simulink subsystem "cabin_suspension"  (R2024a)
settings: Solver=VariableStepAuto  StartTime=0.0  StopTime=10.0  RelTol=1e-3
model mask{Cabin=0}
  mask prompts: Cabin "Cabin Structure"
undefined symbols (not defined in the file or in its folder): cabin, X, Y, Z
libraries: sm_lib x58, Linkage_Shock x16, nesl_utility x6
(part 1 of 2)
settings Model: Creator=lnicolet  LastModifiedBy=lnicolet

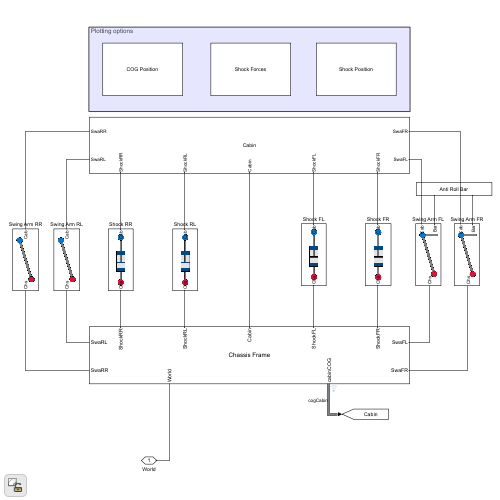
[thumbnail: Simulink's stored preview of the top-level diagram]
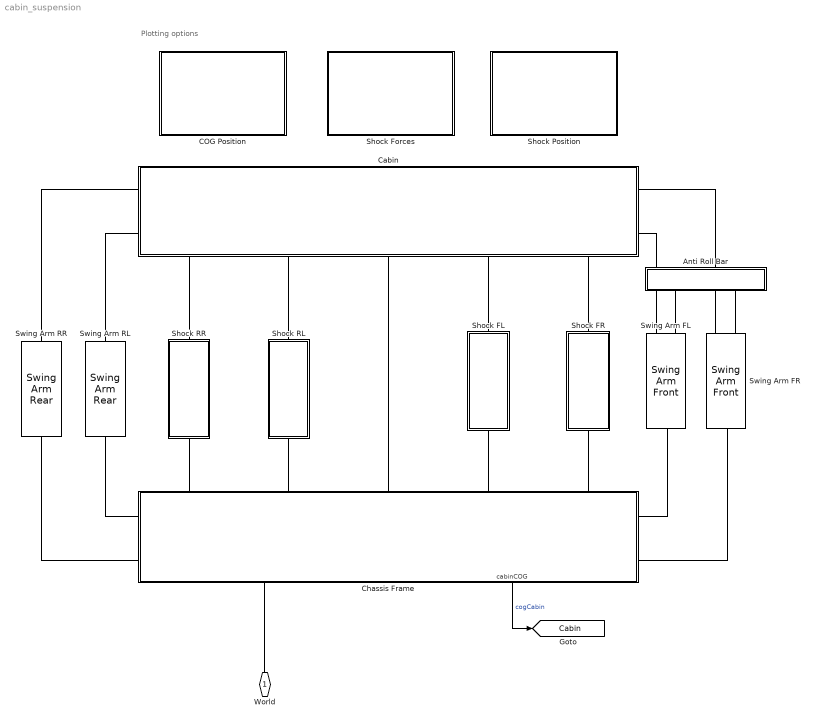
== system cabin_suspension ==
  note: Plotting options
  Anti Roll Bar : Subsystem
      mask Display: disp('Anti Roll Bar')
  COG Position : Subsystem
      settings: OpenFcn=open_system([gcb '/ScopeCabin']);
      mask Display: disp(get_param(gcb,'Name'));
  Cabin : Subsystem
      settings: PortSchema="{\"entries\":[{\"content\":{\"sides\":[{\"content\":{\"connectorIds\":[\"LConn1\",\"LConn2\",\"LConn3\",\"LConn4\",\"LConn5\"]},\"type\":\"ConnectorPlacement.EquallySpacedRectSide\",\"uuid\":\"6c0efb9e-4a15-48d1-a90e-3b8f0520f2fd\"},{\"content\":{\"side\":\"RIGHT\"},\"type\":\"ConnectorPlacement.EquallySpacedRectSide\",\"uuid\":\"c217d90d-c40d-4ab7-8a87-2d7ec4aa75e8\"},{\"content\":{\"connectorIds\":[\"LConn6\",\"LConn7\"],\"side\":\"TOP\"},\"type\":\"ConnectorPlacement.EquallySpacedRectSide\",\"uuid\":\"e70bcc4a-6e95-4530-acee-0e4d1d7170c9\"},{\"content\":{\"connectorIds\":[\"RConn1\",\"RConn2\"],\"side\":\"BOTTOM\"},\"type\":\"ConnectorPlacement.EquallySpacedRectSide\",\"uuid\":\"e953e9a5-e06d-4065-9a29-f0cb41beaf16\"}]},\"type\":\"ConnectorPlacement.EquallySpacedConnector\",\"uuid\":\"c2f1b22e-1df9-453e-a91c-ba57c0256ad1\"}],\"packageUris\":[\"http://schema.mathworks.com/mf0/Connector/R2020b\"],\"version\":\"1.0\"}"
      mask Display: disp('Cabin')
  Chassis Frame : Subsystem
      settings: PortSchema="{\"entries\":[{\"content\":{\"sides\":[{\"content\":{\"connectorIds\":[\"LConn1\",\"Out1\"]},\"type\":\"ConnectorPlacement.EquallySpacedRectSide\",\"uuid\":\"610582a1-14fe-470e-94e3-1e2f1f95b51e\"},{\"content\":{\"connectorIds\":[\"RConn1\",\"RConn2\",\"RConn3\",\"RConn4\",\"RConn5\"],\"side\":\"RIGHT\"},\"type\":\"ConnectorPlacement.EquallySpacedRectSide\",\"uuid\":\"a77f2f37-ea81-4a54-9e68-b60d989bebab\"},{\"content\":{\"connectorIds\":[\"LConn2\",\"LConn3\"],\"side\":\"TOP\"},\"type\":\"ConnectorPlacement.EquallySpacedRectSide\",\"uuid\":\"50ec98b4-a561-4ba0-8e8b-a43aa9d2b054\"},{\"content\":{\"connectorIds\":[\"RConn6\",\"RConn7\"],\"side\":\"BOTTOM\"},\"type\":\"ConnectorPlacement.EquallySpacedRectSide\",\"uuid\":\"9dd61552-a50f-4419-91a1-3a5b07471613\"}]},\"type\":\"ConnectorPlacement.EquallySpacedConnector\",\"uuid\":\"113db540-2e6d-4d54-be76-d99676ae8778\"}],\"packageUris\":[\"http://schema.mathworks.com/mf0/Connector/R2020b\"],\"version\":\"1.0\"}"
      mask Display: disp('Chassis Frame')
  Shock FL : Subsystem
      mask Display: image('Shock_Assembly_IMAGE.png');
  Shock FR : Subsystem
      mask Display: image('Shock_Assembly_IMAGE.png');
  Shock Forces : Subsystem
      settings: OpenFcn=open_system([gcb '/ScopeForces']);
      mask Display: disp(get_param(gcb,'Name'));
  Shock Position : Subsystem
      settings: OpenFcn=open_system([gcb '/ScopeDef']);
      mask Display: disp(get_param(gcb,'Name'));
  Shock RL : Subsystem
      mask Display: image('Shock_Assembly_IMAGE.png');
  Shock RR : Subsystem
      mask Display: image('Shock_Assembly_IMAGE.png');
  Swing Arm FL : Linkage_Shock/Swing Arm Front  posCab=cabin.swingArmCabFL  posCha=cabin.swingArmChasFL  azimuth=cabin.azimuthFL  elevation=cabin.elevationFL
  Swing Arm FR : Linkage_Shock/Swing Arm Front  posCab=cabin.swingArmCabFR  posCha=cabin.swingArmChasFR  azimuth=cabin.azimuthFR  elevation=cabin.elevationFR
  Swing Arm RL : Linkage_Shock/Swing Arm Rear  posCab=cabin.swingArmCabRL  posCha=cabin.swingArmChasRL
  Swing Arm RR : Linkage_Shock/Swing Arm Rear  posCab=cabin.swingArmCabRR  posCha=cabin.swingArmChasRR
  World : PMIOPort  Side=Left
  tag scope: Cabin=global
  wires:
  Chassis Frame/1(cabinCOG) -> [Cabin]  "cogCabin"
  connections:
  Cabin/LConn2 -- Shock RL/RConn1
  Swing Arm RL/LConn1 -- Chassis Frame/LConn3
  World/RConn1 -- Chassis Frame/LConn1
  Swing Arm FR/LConn1 -- Chassis Frame/RConn6
  Chassis Frame/RConn3 -- Cabin/LConn3
  Cabin/LConn1 -- Shock RR/RConn1
  Swing Arm FL/LConn1 -- Chassis Frame/RConn7
  Swing Arm FL/RConn1 -- Cabin/RConn1
  Cabin/LConn4 -- Shock FL/RConn1
  Swing Arm FR/RConn1 -- Cabin/RConn2
  Chassis Frame/LConn2 -- Swing Arm RR/LConn1
  Chassis Frame/RConn4 -- Shock FL/LConn1
  Swing Arm RR/RConn1 -- Cabin/LConn7
  Chassis Frame/RConn5 -- Shock FR/LConn1
  Swing Arm RL/RConn1 -- Cabin/LConn6
  Cabin/LConn5 -- Shock FR/RConn1
  Swing Arm FL/RConn2 -- Anti Roll Bar/LConn1
  Chassis Frame/RConn2 -- Shock RL/LConn1
  Chassis Frame/RConn1 -- Shock RR/LConn1
  Swing Arm FR/RConn2 -- Anti Roll Bar/LConn2

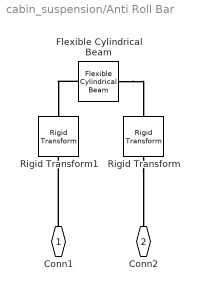
== system cabin_suspension/Anti Roll Bar ==
  Flexible Cylindrical Beam : sm_lib/Body Elements/Flexible Bodies/Beams/Flexible Cylindrical Beam  SectionType=Hollow  Radius=cabin.antiRollBarRadiusOut  RadiusUnits=m  Thickness=cabin.antiRollBarRadiusOut-cabin.antiRollBarRadiusInn  ThicknessUnits=m  Length=norm(cabin.swingArmCabFR-cabin.swingArmCabFL);  LengthUnits=m  StiffnessAndInertiaType=CalculateFromGeometry  Density=cabin.antiRollBarDensity  DensityUnits=kg/m^3  ModuliType=YoungsPoissons  YoungsModulus=cabin.antiRollBarEModulus  YoungsModulusUnits=GPa  PoissonsRatio=cabin.antiRollBarPoisson  ShearModulus=26  ShearModulusUnits=GPa  GeometricCentroid=[0 0]  GeometricCentroidUnits=m  BendingCentroid=[0 0]  BendingCentroidUnits=m  ShearCenter=[0 0]  ShearCenterUnits=m  AxialRigidity=1  AxialRigidityUnits=Pa*m^2  FlexuralRigidity=[1 1]  FlexuralRigidityUnits=Pa*m^4  CrossFlexuralRigidity=0  CrossFlexuralRigidityUnits=Pa*m^4  TorsionalRigidity=1  TorsionalRigidityUnits=Pa*m^4  CenterOfMass=[0 0]  CenterOfMassUnits=m  MassPerUnitLength=1  MassPerUnitLengthUnits=kg/m  MassMomentOfInertiaDensity=[1 1]  MassMomentOfInertiaDensityUnits=kg*m  MassProductOfInertiaDensity=0  MassProductOfInertiaDensityUnits=kg*m  DampingType=Proportional  ProportionalDampingAlpha=0  ProportionalDampingAlphaUnits=1/s  ProportionalDampingBeta=0.001  ProportionalDampingBetaUnits=s  UniformModalDampingRatio=0.01  NumElements=1  ReductionType=None  NumRetainedModes=1  GraphicType=FromGeometry  GraphicVisPropType=SimpleVisualProperties  GraphicDiffuseColor=[0.5 0.5 0.5]  GraphicOpacity=1  GraphicSpecularColor=[0.5 0.5 0.5 1.0]  GraphicAmbientColor=[0.15 0.15 0.15 1.0]  GraphicEmissiveColor=[0.0 0.0 0.0 1.0]  GraphicShininess=75  DoExposeZminFrame=on  DoExposeZmaxFrame=on  SerializedFrames=<Frames/>
  Rigid Transform : sm_lib/Frames and Transforms/Rigid Transform  RotationMethod=StandardAxis  FollAlignAxisA=+X  BaseAlignAxisA=+Y  FollAlignAxisB=+Y  BaseAlignAxisB=+Z  RotationStandardAxis=+X  RotationAngle=90  RotationAngleUnits=deg  RotationArbitraryAxis=[0 0 1]  RotationSequenceAxes=FollowerAxes  RotationSequence=XYX  RotationSequenceAngles=[0 0 0]  RotationSequenceAnglesUnits=deg  RotationMatrix=[1 0 0;0 1 0;0 0 1]  Quaternion=[1 0 0 0]  TranslationMethod=None  TranslationCartesianOffset=[0 0 0]  TranslationCartesianOffsetUnits=m  TranslationStandardAxis=+Z  TranslationStandardOffset=0  TranslationStandardOffsetUnits=m  TranslationROffset=0  TranslationROffsetUnits=m  TranslationThetaOffset=0  TranslationThetaOffsetUnits=deg  TranslationZOffset=0  TranslationZOffsetUnits=m
  Rigid Transform1 : sm_lib/Frames and Transforms/Rigid Transform  RotationMethod=StandardAxis  FollAlignAxisA=+X  BaseAlignAxisA=+Y  FollAlignAxisB=+Y  BaseAlignAxisB=+Z  RotationStandardAxis=+X  RotationAngle=90  RotationAngleUnits=deg  RotationArbitraryAxis=[0 0 1]  RotationSequenceAxes=FollowerAxes  RotationSequence=XYX  RotationSequenceAngles=[0 0 0]  RotationSequenceAnglesUnits=deg  RotationMatrix=[1 0 0;0 1 0;0 0 1]  Quaternion=[1 0 0 0]  TranslationMethod=None  TranslationCartesianOffset=[0 0 0]  TranslationCartesianOffsetUnits=m  TranslationStandardAxis=+Z  TranslationStandardOffset=0  TranslationStandardOffsetUnits=m  TranslationROffset=0  TranslationROffsetUnits=m  TranslationThetaOffset=0  TranslationThetaOffsetUnits=deg  TranslationZOffset=0  TranslationZOffsetUnits=m
  Conn1 : PMIOPort  Side=Left
  Conn2 : PMIOPort  Port=2  Side=Left
  connections:
  Conn1/RConn1 -- Rigid Transform1/LConn1
  Flexible Cylindrical Beam/RConn1 -- Rigid Transform/RConn1
  Rigid Transform/LConn1 -- Conn2/RConn1
  Flexible Cylindrical Beam/LConn1 -- Rigid Transform1/RConn1

== system cabin_suspension/COG Position ==
  Bus Selector : BusSelector  OutputSignals=px,py,pz,angx,angy,angz
  ScopeCabin : Scope  NumInputPorts=6
  wires:
  Bus Selector/6 -> ScopeCabin/6  "<angz>"
  Bus Selector/5 -> ScopeCabin/5  "<angy>"
  Bus Selector/4 -> ScopeCabin/4  "<angx>"
  Bus Selector/3 -> ScopeCabin/3  "<pz>"
  Bus Selector/2 -> ScopeCabin/2  "<py>"
  Bus Selector/1 -> ScopeCabin/1  "<px>"
  [Cabin] -> Bus Selector/1

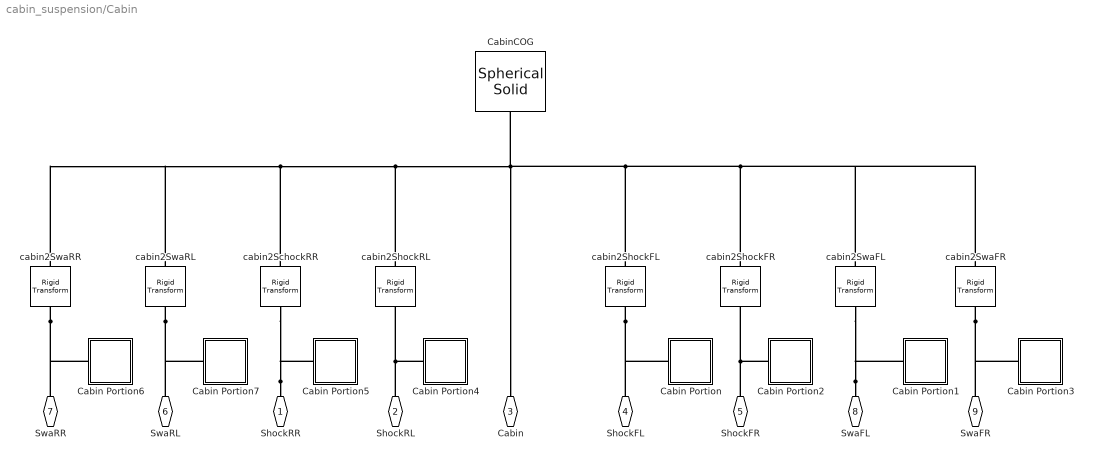
== system cabin_suspension/Cabin ==
  Cabin Portion : Subsystem
  Cabin Portion1 : Subsystem
  Cabin Portion2 : Subsystem
  Cabin Portion3 : Subsystem
  Cabin Portion4 : Subsystem
  Cabin Portion5 : Subsystem
  Cabin Portion6 : Subsystem
  Cabin Portion7 : Subsystem
  CabinCOG : sm_lib/Body Elements/Spherical Solid  SphereRadius=0.03  SphereRadiusUnits=m  ExportEntireGeometry=off  InertiaType=Custom  BasedOnType=Mass  Density=1000  DensityUnits=kg/m^3  Mass=cabin.cabinMass  MassUnits=kg  CenterOfMass=[0 0 0]  CenterOfMassUnits=m  MomentsOfInertia=[cabin.cabinJxx,cabin.cabinJyy,cabin.cabinJzz]  MomentsOfInertiaUnits=kg*m^2  ProductsOfInertia=[0 0 0]  ProductsOfInertiaUnits=kg*m^2  GraphicType=FromGeometry  MarkerShape=Sphere  MarkerSize=10  GraphicVisPropType=SimpleVisualProperties  GraphicDiffuseColor=[0,0,1]  GraphicOpacity=1  GraphicSpecularColor=[0.5 0.5 0.5 1.0]  GraphicAmbientColor=[0.15 0.15 0.15 1.0]  GraphicEmissiveColor=[0.0 0.0 0.0 1.0]  GraphicShininess=75  DoExposeReferenceFrame=on  SerializedFrames=<Frames/>
  cabin2SchockRR : sm_lib/Frames and Transforms/Rigid Transform  RotationMethod=None  FollAlignAxisA=+X  BaseAlignAxisA=+Y  FollAlignAxisB=+Y  BaseAlignAxisB=+Z  RotationStandardAxis=+Z  RotationAngle=0  RotationAngleUnits=deg  RotationArbitraryAxis=[0 0 1]  RotationSequenceAxes=FollowerAxes  RotationSequence=XYX  RotationSequenceAngles=[0 0 0]  RotationSequenceAnglesUnits=deg  RotationMatrix=[1 0 0;0 1 0;0 0 1]  Quaternion=[1 0 0 0]  TranslationMethod=Cartesian  TranslationCartesianOffset=cabin.schockTopPosRR-cabin.cabinOriginStart  TranslationCartesianOffsetUnits=m  TranslationStandardAxis=+Z  TranslationStandardOffset=0  TranslationStandardOffsetUnits=m  TranslationROffset=0  TranslationROffsetUnits=m  TranslationThetaOffset=0  TranslationThetaOffsetUnits=deg  TranslationZOffset=0  TranslationZOffsetUnits=m
  cabin2ShockFL : sm_lib/Frames and Transforms/Rigid Transform  RotationMethod=None  FollAlignAxisA=+X  BaseAlignAxisA=+Y  FollAlignAxisB=+Y  BaseAlignAxisB=+Z  RotationStandardAxis=+Z  RotationAngle=0  RotationAngleUnits=deg  RotationArbitraryAxis=[0 0 1]  RotationSequenceAxes=FollowerAxes  RotationSequence=XYX  RotationSequenceAngles=[0 0 0]  RotationSequenceAnglesUnits=deg  RotationMatrix=[1 0 0;0 1 0;0 0 1]  Quaternion=[1 0 0 0]  TranslationMethod=Cartesian  TranslationCartesianOffset=cabin.schockTopPosFL-cabin.cabinOriginStart  TranslationCartesianOffsetUnits=m  TranslationStandardAxis=+Z  TranslationStandardOffset=0  TranslationStandardOffsetUnits=m  TranslationROffset=0  TranslationROffsetUnits=m  TranslationThetaOffset=0  TranslationThetaOffsetUnits=deg  TranslationZOffset=0  TranslationZOffsetUnits=m
  cabin2ShockFR : sm_lib/Frames and Transforms/Rigid Transform  RotationMethod=None  FollAlignAxisA=+X  BaseAlignAxisA=+Y  FollAlignAxisB=+Y  BaseAlignAxisB=+Z  RotationStandardAxis=+Z  RotationAngle=0  RotationAngleUnits=deg  RotationArbitraryAxis=[0 0 1]  RotationSequenceAxes=FollowerAxes  RotationSequence=XYX  RotationSequenceAngles=[0 0 0]  RotationSequenceAnglesUnits=deg  RotationMatrix=[1 0 0;0 1 0;0 0 1]  Quaternion=[1 0 0 0]  TranslationMethod=Cartesian  TranslationCartesianOffset=cabin.schockTopPosFR-cabin.cabinOriginStart  TranslationCartesianOffsetUnits=m  TranslationStandardAxis=+Z  TranslationStandardOffset=0  TranslationStandardOffsetUnits=m  TranslationROffset=0  TranslationROffsetUnits=m  TranslationThetaOffset=0  TranslationThetaOffsetUnits=deg  TranslationZOffset=0  TranslationZOffsetUnits=m
  cabin2ShockRL : sm_lib/Frames and Transforms/Rigid Transform  RotationMethod=None  FollAlignAxisA=+X  BaseAlignAxisA=+Y  FollAlignAxisB=+Y  BaseAlignAxisB=+Z  RotationStandardAxis=+Z  RotationAngle=0  RotationAngleUnits=deg  RotationArbitraryAxis=[0 0 1]  RotationSequenceAxes=FollowerAxes  RotationSequence=XYX  RotationSequenceAngles=[0 0 0]  RotationSequenceAnglesUnits=deg  RotationMatrix=[1 0 0;0 1 0;0 0 1]  Quaternion=[1 0 0 0]  TranslationMethod=Cartesian  TranslationCartesianOffset=cabin.schockTopPosRL-cabin.cabinOriginStart  TranslationCartesianOffsetUnits=m  TranslationStandardAxis=+Z  TranslationStandardOffset=0  TranslationStandardOffsetUnits=m  TranslationROffset=0  TranslationROffsetUnits=m  TranslationThetaOffset=0  TranslationThetaOffsetUnits=deg  TranslationZOffset=0  TranslationZOffsetUnits=m
  cabin2SwaFL : sm_lib/Frames and Transforms/Rigid Transform  RotationMethod=None  FollAlignAxisA=+X  BaseAlignAxisA=+Y  FollAlignAxisB=+Y  BaseAlignAxisB=+Z  RotationStandardAxis=+X  RotationAngle=-90  RotationAngleUnits=deg  RotationArbitraryAxis=[0 0 1]  RotationSequenceAxes=FollowerAxes  RotationSequence=XYX  RotationSequenceAngles=[0 0 0]  RotationSequenceAnglesUnits=deg  RotationMatrix=[1 0 0;0 1 0;0 0 1]  Quaternion=[1 0 0 0]  TranslationMethod=Cartesian  TranslationCartesianOffset=cabin.swingArmCabFL-cabin.cabinOriginStart  TranslationCartesianOffsetUnits=m  TranslationStandardAxis=+Z  TranslationStandardOffset=0  TranslationStandardOffsetUnits=m  TranslationROffset=0  TranslationROffsetUnits=m  TranslationThetaOffset=0  TranslationThetaOffsetUnits=deg  TranslationZOffset=0  TranslationZOffsetUnits=m
  cabin2SwaFR : sm_lib/Frames and Transforms/Rigid Transform  RotationMethod=None  FollAlignAxisA=+X  BaseAlignAxisA=+Y  FollAlignAxisB=+Y  BaseAlignAxisB=+Z  RotationStandardAxis=+X  RotationAngle=-90  RotationAngleUnits=deg  RotationArbitraryAxis=[0 0 1]  RotationSequenceAxes=FollowerAxes  RotationSequence=XYX  RotationSequenceAngles=[0 0 0]  RotationSequenceAnglesUnits=deg  RotationMatrix=[1 0 0;0 1 0;0 0 1]  Quaternion=[1 0 0 0]  TranslationMethod=Cartesian  TranslationCartesianOffset=cabin.swingArmCabFR-cabin.cabinOriginStart  TranslationCartesianOffsetUnits=m  TranslationStandardAxis=+Z  TranslationStandardOffset=0  TranslationStandardOffsetUnits=m  TranslationROffset=0  TranslationROffsetUnits=m  TranslationThetaOffset=0  TranslationThetaOffsetUnits=deg  TranslationZOffset=0  TranslationZOffsetUnits=m
  cabin2SwaRL : sm_lib/Frames and Transforms/Rigid Transform  RotationMethod=None  FollAlignAxisA=+X  BaseAlignAxisA=+Y  FollAlignAxisB=+Y  BaseAlignAxisB=+Z  RotationStandardAxis=+X  RotationAngle=-90  RotationAngleUnits=deg  RotationArbitraryAxis=[0 0 1]  RotationSequenceAxes=FollowerAxes  RotationSequence=XYX  RotationSequenceAngles=[0 0 0]  RotationSequenceAnglesUnits=deg  RotationMatrix=[1 0 0;0 1 0;0 0 1]  Quaternion=[1 0 0 0]  TranslationMethod=Cartesian  TranslationCartesianOffset=cabin.swingArmCabRL-cabin.cabinOriginStart  TranslationCartesianOffsetUnits=m  TranslationStandardAxis=+Z  TranslationStandardOffset=0  TranslationStandardOffsetUnits=m  TranslationROffset=0  TranslationROffsetUnits=m  TranslationThetaOffset=0  TranslationThetaOffsetUnits=deg  TranslationZOffset=0  TranslationZOffsetUnits=m
  cabin2SwaRR : sm_lib/Frames and Transforms/Rigid Transform  RotationMethod=None  FollAlignAxisA=+X  BaseAlignAxisA=+Y  FollAlignAxisB=+Y  BaseAlignAxisB=+Z  RotationStandardAxis=+X  RotationAngle=-90  RotationAngleUnits=deg  RotationArbitraryAxis=[0 0 1]  RotationSequenceAxes=FollowerAxes  RotationSequence=XYX  RotationSequenceAngles=[0 0 0]  RotationSequenceAnglesUnits=deg  RotationMatrix=[1 0 0;0 1 0;0 0 1]  Quaternion=[1 0 0 0]  TranslationMethod=Cartesian  TranslationCartesianOffset=cabin.swingArmCabRR-cabin.cabinOriginStart  TranslationCartesianOffsetUnits=m  TranslationStandardAxis=+Z  TranslationStandardOffset=0  TranslationStandardOffsetUnits=m  TranslationROffset=0  TranslationROffsetUnits=m  TranslationThetaOffset=0  TranslationThetaOffsetUnits=deg  TranslationZOffset=0  TranslationZOffsetUnits=m
  ShockRR : PMIOPort  Side=Left
  ShockRL : PMIOPort  Port=2  Side=Left
  Cabin : PMIOPort  Port=3  Side=Left
  ShockFL : PMIOPort  Port=4  Side=Left
  ShockFR : PMIOPort  Port=5  Side=Left
  SwaRL : PMIOPort  Port=6  Side=Left
  SwaRR : PMIOPort  Port=7  Side=Left
  SwaFL : PMIOPort  Port=8  Side=Right
  SwaFR : PMIOPort  Port=9  Side=Right
  connections:
  SwaFL/RConn1 -- Cabin Portion1/LConn1 -- cabin2SwaFL/RConn1
  cabin2SwaFR/RConn1 -- Cabin Portion3/LConn1 -- SwaFR/RConn1
  cabin2ShockFL/RConn1 -- Cabin Portion/LConn1 -- ShockFL/RConn1
  cabin2SwaRR/RConn1 -- Cabin Portion6/LConn1 -- SwaRR/RConn1
  ShockRR/RConn1 -- Cabin Portion5/LConn1 -- cabin2SchockRR/RConn1
  cabin2SwaRL/RConn1 -- Cabin Portion7/LConn1 -- SwaRL/RConn1
  Cabin Portion2/LConn1 -- cabin2ShockFR/RConn1 -- ShockFR/RConn1
  Cabin Portion4/LConn1 -- cabin2ShockRL/RConn1 -- ShockRL/RConn1
  cabin2ShockFL/LConn1 -- cabin2SchockRR/LConn1 -- cabin2SwaRR/LConn1 -- cabin2SwaRL/LConn1 -- cabin2ShockRL/LConn1 -- Cabin/RConn1 -- CabinCOG/RConn1 -- cabin2ShockFR/LConn1 -- cabin2SwaFR/LConn1 -- cabin2SwaFL/LConn1

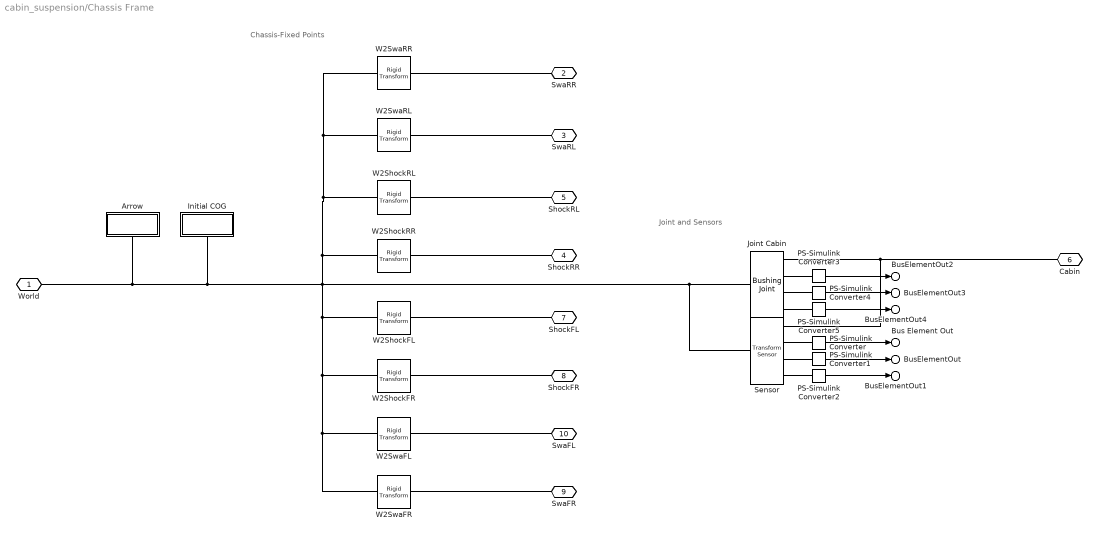
== system cabin_suspension/Chassis Frame ==
  note: Joint and Sensors
  note: Chassis-Fixed Points
  Arrow : Subsystem
      mask Display: disp(get_param(gcb,'Name'));
  Initial COG : Subsystem
      mask Display: disp(get_param(gcb,'Name'));
  Joint Cabin : sm_lib/Joints/Bushing Joint  JointMode=Normal  CompositeWrenchDir=FollowerOnBase  CompositeWrenchFrame=BaseFrame  SenseConstraintForce=off  SenseConstraintTorque=off  SenseTotalForce=off  SenseTotalTorque=off  PxPositionTargetSpecify=on  PxPositionTargetPriority=High  PxPositionTargetValue=cabin.cabinOriginStart(1)  PxPositionTargetValueUnits=m  PxVelocityTargetSpecify=off  PxVelocityTargetPriority=High  PxVelocityTargetValue=0  PxVelocityTargetValueUnits=m/s  PxEquilibriumPosition=0  PxEquilibriumPositionUnits=m  PxSpringStiffness=0  PxSpringStiffnessUnits=N/m  PxDampingCoefficient=0  PxDampingCoefficientUnits=N/(m/s)  PxLowerLimitSpecify=off  PxLowerLimitBound=-1  PxLowerLimitBoundUnits=m  PxLowerLimitStiffness=1e6  PxLowerLimitStiffnessUnits=N/m  PxLowerLimitDamping=1e3  PxLowerLimitDampingUnits=N/(m/s)  PxLowerLimitTransitionRegionWidth=1e-4  PxLowerLimitTransitionRegionWidthUnits=m  PxUpperLimitSpecify=off  PxUpperLimitBound=1  PxUpperLimitBoundUnits=m  PxUpperLimitStiffness=1e6  PxUpperLimitStiffnessUnits=N/m  PxUpperLimitDamping=1e3  PxUpperLimitDampingUnits=N/(m/s)  PxUpperLimitTransitionRegionWidth=1e-4  PxUpperLimitTransitionRegionWidthUnits=m  PxTorqueActuationMode=NoTorque  PxMotionActuationMode=ComputedMotion  PxSensePosition=off  PxSenseVelocity=off  PxSenseAcceleration=off  PxSenseTorqueForce=off  PxSenseLowerLimitTorqueForce=off  PxSenseUpperLimitTorqueForce=off  PyPositionTargetSpecify=on  PyPositionTargetPriority=High  PyPositionTargetValue=cabin.cabinOriginStart(2)  PyPositionTargetValueUnits=m  PyVelocityTargetSpecify=off  PyVelocityTargetPriority=High  PyVelocityTargetValue=0  PyVelocityTargetValueUnits=m/s  PyEquilibriumPosition=0  PyEquilibriumPositionUnits=m  PySpringStiffness=0  PySpringStiffnessUnits=N/m  PyDampingCoefficient=0  PyDampingCoefficientUnits=N/(m/s)  PyLowerLimitSpecify=off  PyLowerLimitBound=-1  PyLowerLimitBoundUnits=m  PyLowerLimitStiffness=1e6  PyLowerLimitStiffnessUnits=N/m  PyLowerLimitDamping=1e3  PyLowerLimitDampingUnits=N/(m/s)  PyLowerLimitTransitionRegionWidth=1e-4  PyLowerLimitTransitionRegionWidthUnits=m  PyUpperLimitSpecify=off  PyUpperLimitBound=1  PyUpperLimitBoundUnits=m  PyUpperLimitStiffness=1e6  PyUpperLimitStiffnessUnits=N/m  PyUpperLimitDamping=1e3  PyUpperLimitDampingUnits=N/(m/s)  PyUpperLimitTransitionRegionWidth=1e-4  PyUpperLimitTransitionRegionWidthUnits=m  PyTorqueActuationMode=NoTorque  PyMotionActuationMode=ComputedMotion  PySensePosition=off  PySenseVelocity=off  PySenseAcceleration=off  PySenseTorqueForce=off  PySenseLowerLimitTorqueForce=off  PySenseUpperLimitTorqueForce=off  PzPositionTargetSpecify=on  PzPositionTargetPriority=High  PzPositionTargetValue=cabin.cabinOriginStart(3)  PzPositionTargetValueUnits=m  PzVelocityTargetSpecify=off  PzVelocityTargetPriority=High  PzVelocityTargetValue=0  PzVelocityTargetValueUnits=m/s  PzEquilibriumPosition=0  PzEquilibriumPositionUnits=m  PzSpringStiffness=0  PzSpringStiffnessUnits=N/m  PzDampingCoefficient=0  PzDampingCoefficientUnits=N/(m/s)  PzLowerLimitSpecify=off  PzLowerLimitBound=-1  PzLowerLimitBoundUnits=m  PzLowerLimitStiffness=1e6  PzLowerLimitStiffnessUnits=N/m  PzLowerLimitDamping=1e3  PzLowerLimitDampingUnits=N/(m/s)  PzLowerLimitTransitionRegionWidth=1e-4  PzLowerLimitTransitionRegionWidthUnits=m  PzUpperLimitSpecify=off  PzUpperLimitBound=1  PzUpperLimitBoundUnits=m  PzUpperLimitStiffness=1e6  PzUpperLimitStiffnessUnits=N/m  PzUpperLimitDamping=1e3  PzUpperLimitDampingUnits=N/(m/s)  PzUpperLimitTransitionRegionWidth=1e-4  PzUpperLimitTransitionRegionWidthUnits=m  PzTorqueActuationMode=NoTorque  PzMotionActuationMode=ComputedMotion  PzSensePosition=off  PzSenseVelocity=off  PzSenseAcceleration=off  PzSenseTorqueForce=off  PzSenseLowerLimitTorqueForce=off  PzSenseUpperLimitTorqueForce=off  RxPositionTargetSpecify=on  RxPositionTargetPriority=High  RxPositionTargetValue=0  RxPositionTargetValueUnits=deg  RxVelocityTargetSpecify=off  RxVelocityTargetPriority=High  RxVelocityTargetValue=0  RxVelocityTargetValueUnits=deg/s  RxEquilibriumPosition=0  RxEquilibriumPositionUnits=deg  RxSpringStiffness=0  RxSpringStiffnessUnits=N*m/deg  RxDampingCoefficient=0  RxDampingCoefficientUnits=N*m/(deg/s)  RxLowerLimitSpecify=off  RxLowerLimitBound=-90  RxLowerLimitBoundUnits=deg  RxLowerLimitStiffness=1e4  RxLowerLimitStiffnessUnits=N*m/deg  RxLowerLimitDamping=10  RxLowerLimitDampingUnits=N*m/(deg/s)  RxLowerLimitTransitionRegionWidth=0.1  RxLowerLimitTransitionRegionWidthUnits=deg  RxUpperLimitSpecify=off  RxUpperLimitBound=90  RxUpperLimitBoundUnits=deg  RxUpperLimitStiffness=1e4  RxUpperLimitStiffnessUnits=N*m/deg  RxUpperLimitDamping=10  RxUpperLimitDampingUnits=N*m/(deg/s)  RxUpperLimitTransitionRegionWidth=0.1  RxUpperLimitTransitionRegionWidthUnits=deg  RxTorqueActuationMode=NoTorque  RxMotionActuationMode=ComputedMotion  RxSensePosition=on  RxSenseVelocity=off  RxSenseAcceleration=off  RxSenseTorqueForce=off  RxSenseLowerLimitTorqueForce=off  RxSenseUpperLimitTorqueForce=off  RyPositionTargetSpecify=on  RyPositionTargetPriority=High  RyPositionTargetValue=0  RyPositionTargetValueUnits=deg  RyVelocityTargetSpecify=off  RyVelocityTargetPriority=High  RyVelocityTargetValue=0  RyVelocityTargetValueUnits=deg/s  RyEquilibriumPosition=0  RyEquilibriumPositionUnits=deg  RySpringStiffness=0  RySpringStiffnessUnits=N*m/deg  RyDampingCoefficient=0  RyDampingCoefficientUnits=N*m/(deg/s)  RyLowerLimitSpecify=off  RyLowerLimitBound=-90  RyLowerLimitBoundUnits=deg  RyLowerLimitStiffness=1e4  RyLowerLimitStiffnessUnits=N*m/deg  RyLowerLimitDamping=10  RyLowerLimitDampingUnits=N*m/(deg/s)  RyLowerLimitTransitionRegionWidth=0.1  RyLowerLimitTransitionRegionWidthUnits=deg  RyUpperLimitSpecify=off  RyUpperLimitBound=90  RyUpperLimitBoundUnits=deg  RyUpperLimitStiffness=1e4  RyUpperLimitStiffnessUnits=N*m/deg  RyUpperLimitDamping=10  RyUpperLimitDampingUnits=N*m/(deg/s)  RyUpperLimitTransitionRegionWidth=0.1  RyUpperLimitTransitionRegionWidthUnits=deg  RyTorqueActuationMode=NoTorque  RyMotionActuationMode=ComputedMotion  RySensePosition=on  RySenseVelocity=off  RySenseAcceleration=off  RySenseTorqueForce=off  RySenseLowerLimitTorqueForce=off  RySenseUpperLimitTorqueForce=off  RzPositionTargetSpecify=on  RzPositionTargetPriority=High  RzPositionTargetValue=0  RzPositionTargetValueUnits=deg  RzVelocityTargetSpecify=off  RzVelocityTargetPriority=High  RzVelocityTargetValue=0  RzVelocityTargetValueUnits=deg/s  RzEquilibriumPosition=0  RzEquilibriumPositionUnits=deg  RzSpringStiffness=0  RzSpringStiffnessUnits=N*m/deg  RzDampingCoefficient=0  RzDampingCoefficientUnits=N*m/(deg/s)  RzLowerLimitSpecify=off  RzLowerLimitBound=-90  RzLowerLimitBoundUnits=deg  RzLowerLimitStiffness=1e4  RzLowerLimitStiffnessUnits=N*m/deg  RzLowerLimitDamping=10  RzLowerLimitDampingUnits=N*m/(deg/s)  RzLowerLimitTransitionRegionWidth=0.1  RzLowerLimitTransitionRegionWidthUnits=deg  RzUpperLimitSpecify=off  RzUpperLimitBound=90  RzUpperLimitBoundUnits=deg  RzUpperLimitStiffness=1e4  RzUpperLimitStiffnessUnits=N*m/deg  RzUpperLimitDamping=10  RzUpperLimitDampingUnits=N*m/(deg/s)  RzUpperLimitTransitionRegionWidth=0.1  RzUpperLimitTransitionRegionWidthUnits=deg  RzTorqueActuationMode=NoTorque  RzMotionActuationMode=ComputedMotion  RzSensePosition=on  RzSenseVelocity=off  RzSenseAcceleration=off  RzSenseTorqueForce=off  RzSenseLowerLimitTorqueForce=off  RzSenseUpperLimitTorqueForce=off
  PS-Simulink Converter : nesl_utility/PS-Simulink Converter  PhysicalDomain=network_engine_domain  SubClassName=ps_output  LeftPortType=input  RightPortType=output  PseudoPeriodic=off  Frequencies=[]  VectorFormat=inherit  Unit=m  AffineConversion=off
  PS-Simulink Converter1 : nesl_utility/PS-Simulink Converter  PhysicalDomain=network_engine_domain  SubClassName=ps_output  LeftPortType=input  RightPortType=output  PseudoPeriodic=off  Frequencies=[]  VectorFormat=inherit  Unit=m  AffineConversion=off
  PS-Simulink Converter2 : nesl_utility/PS-Simulink Converter  PhysicalDomain=network_engine_domain  SubClassName=ps_output  LeftPortType=input  RightPortType=output  PseudoPeriodic=off  Frequencies=[]  VectorFormat=inherit  Unit=m  AffineConversion=off
  PS-Simulink Converter3 : nesl_utility/PS-Simulink Converter  PhysicalDomain=network_engine_domain  SubClassName=ps_output  LeftPortType=input  RightPortType=output  PseudoPeriodic=off  Frequencies=[]  VectorFormat=inherit  Unit=deg  AffineConversion=off
  PS-Simulink Converter4 : nesl_utility/PS-Simulink Converter  PhysicalDomain=network_engine_domain  SubClassName=ps_output  LeftPortType=input  RightPortType=output  PseudoPeriodic=off  Frequencies=[]  VectorFormat=inherit  Unit=deg  AffineConversion=off
  PS-Simulink Converter5 : nesl_utility/PS-Simulink Converter  PhysicalDomain=network_engine_domain  SubClassName=ps_output  LeftPortType=input  RightPortType=output  PseudoPeriodic=off  Frequencies=[]  VectorFormat=inherit  Unit=deg  AffineConversion=off
  "Sensor " : sm_lib/Frames and Transforms/Transform Sensor  MeasurementFrame=World  RotationSequence=XYX  SenseAngle=off  SenseAxis=off  SenseQ=off  SenseR=off  SenseRotationSequence=off  SenseOmegaX=off  SenseOmegaY=off  SenseOmegaZ=off  SenseOmega=off  SenseQDot=off  SenseRDot=off  SenseRotationSequenceDot=off  SenseAlphaX=off  SenseAlphaY=off  SenseAlphaZ=off  SenseAlpha=off  SenseQDDot=off  SenseRDDot=off  SenseX=on  SenseY=on  SenseZ=on  SenseXYZ=off  SenseRad=off  SenseAzim=off  SenseDist=off  SenseInc=off  SenseXDot=off  SenseYDot=off  SenseZDot=off  SenseXYZDot=off  SenseRadDot=off  SenseAzimDot=off  SenseDistDot=off  SenseIncDot=off  SenseXDDot=off  SenseYDDot=off  SenseZDDot=off  SenseXYZDDot=off  SenseRadDDot=off  SenseAzimDDot=off  SenseDistDDot=off  SenseIncDDot=off
  W2ShockFL : sm_lib/Frames and Transforms/Rigid Transform  RotationMethod=None  FollAlignAxisA=+X  BaseAlignAxisA=+Y  FollAlignAxisB=+Y  BaseAlignAxisB=+Z  RotationStandardAxis=+Z  RotationAngle=0  RotationAngleUnits=deg  RotationArbitraryAxis=[0 0 1]  RotationSequenceAxes=FollowerAxes  RotationSequence=XYX  RotationSequenceAngles=[0 0 0]  RotationSequenceAnglesUnits=deg  RotationMatrix=[1 0 0;0 1 0;0 0 1]  Quaternion=[1 0 0 0]  TranslationMethod=Cartesian  TranslationCartesianOffset=cabin.schockBotPosFL  TranslationCartesianOffsetUnits=m  TranslationStandardAxis=+Z  TranslationStandardOffset=0  TranslationStandardOffsetUnits=m  TranslationROffset=0  TranslationROffsetUnits=m  TranslationThetaOffset=0  TranslationThetaOffsetUnits=deg  TranslationZOffset=0  TranslationZOffsetUnits=m
  W2ShockFR : sm_lib/Frames and Transforms/Rigid Transform  RotationMethod=None  FollAlignAxisA=+X  BaseAlignAxisA=+Y  FollAlignAxisB=+Y  BaseAlignAxisB=+Z  RotationStandardAxis=+Z  RotationAngle=0  RotationAngleUnits=deg  RotationArbitraryAxis=[0 0 1]  RotationSequenceAxes=FollowerAxes  RotationSequence=XYX  RotationSequenceAngles=[0 0 0]  RotationSequenceAnglesUnits=deg  RotationMatrix=[1 0 0;0 1 0;0 0 1]  Quaternion=[1 0 0 0]  TranslationMethod=Cartesian  TranslationCartesianOffset=cabin.schockBotPosFR  TranslationCartesianOffsetUnits=m  TranslationStandardAxis=+Z  TranslationStandardOffset=0  TranslationStandardOffsetUnits=m  TranslationROffset=0  TranslationROffsetUnits=m  TranslationThetaOffset=0  TranslationThetaOffsetUnits=deg  TranslationZOffset=0  TranslationZOffsetUnits=m
  W2ShockRL : sm_lib/Frames and Transforms/Rigid Transform  RotationMethod=None  FollAlignAxisA=+X  BaseAlignAxisA=+Y  FollAlignAxisB=+Y  BaseAlignAxisB=+Z  RotationStandardAxis=+Z  RotationAngle=0  RotationAngleUnits=deg  RotationArbitraryAxis=[0 0 1]  RotationSequenceAxes=FollowerAxes  RotationSequence=XYX  RotationSequenceAngles=[0 0 0]  RotationSequenceAnglesUnits=deg  RotationMatrix=[1 0 0;0 1 0;0 0 1]  Quaternion=[1 0 0 0]  TranslationMethod=Cartesian  TranslationCartesianOffset=cabin.schockBotPosRL  TranslationCartesianOffsetUnits=m  TranslationStandardAxis=+Z  TranslationStandardOffset=0  TranslationStandardOffsetUnits=m  TranslationROffset=0  TranslationROffsetUnits=m  TranslationThetaOffset=0  TranslationThetaOffsetUnits=deg  TranslationZOffset=0  TranslationZOffsetUnits=m
  W2ShockRR : sm_lib/Frames and Transforms/Rigid Transform  RotationMethod=None  FollAlignAxisA=+X  BaseAlignAxisA=+Y  FollAlignAxisB=+Y  BaseAlignAxisB=+Z  RotationStandardAxis=+Z  RotationAngle=0  RotationAngleUnits=deg  RotationArbitraryAxis=[0 0 1]  RotationSequenceAxes=FollowerAxes  RotationSequence=XYX  RotationSequenceAngles=[0 0 0]  RotationSequenceAnglesUnits=deg  RotationMatrix=[1 0 0;0 1 0;0 0 1]  Quaternion=[1 0 0 0]  TranslationMethod=Cartesian  TranslationCartesianOffset=cabin.schockBotPosRR  TranslationCartesianOffsetUnits=m  TranslationStandardAxis=+Z  TranslationStandardOffset=0  TranslationStandardOffsetUnits=m  TranslationROffset=0  TranslationROffsetUnits=m  TranslationThetaOffset=0  TranslationThetaOffsetUnits=deg  TranslationZOffset=0  TranslationZOffsetUnits=m
  W2SwaFL : sm_lib/Frames and Transforms/Rigid Transform  RotationMethod=None  FollAlignAxisA=+X  BaseAlignAxisA=+Y  FollAlignAxisB=+Y  BaseAlignAxisB=+Z  RotationStandardAxis=+X  RotationAngle=-90  RotationAngleUnits=deg  RotationArbitraryAxis=[0 0 1]  RotationSequenceAxes=FollowerAxes  RotationSequence=XYX  RotationSequenceAngles=[0 0 0]  RotationSequenceAnglesUnits=deg  RotationMatrix=[1 0 0;0 1 0;0 0 1]  Quaternion=[1 0 0 0]  TranslationMethod=Cartesian  TranslationCartesianOffset=cabin.swingArmChasFL  TranslationCartesianOffsetUnits=m  TranslationStandardAxis=+Z  TranslationStandardOffset=0  TranslationStandardOffsetUnits=m  TranslationROffset=0  TranslationROffsetUnits=m  TranslationThetaOffset=0  TranslationThetaOffsetUnits=deg  TranslationZOffset=0  TranslationZOffsetUnits=m
  W2SwaFR : sm_lib/Frames and Transforms/Rigid Transform  RotationMethod=None  FollAlignAxisA=+X  BaseAlignAxisA=+Y  FollAlignAxisB=+Y  BaseAlignAxisB=+Z  RotationStandardAxis=+X  RotationAngle=-90  RotationAngleUnits=deg  RotationArbitraryAxis=[0 0 1]  RotationSequenceAxes=FollowerAxes  RotationSequence=XYX  RotationSequenceAngles=[0 0 0]  RotationSequenceAnglesUnits=deg  RotationMatrix=[1 0 0;0 1 0;0 0 1]  Quaternion=[1 0 0 0]  TranslationMethod=Cartesian  TranslationCartesianOffset=cabin.swingArmChasFR  TranslationCartesianOffsetUnits=m  TranslationStandardAxis=+Z  TranslationStandardOffset=0  TranslationStandardOffsetUnits=m  TranslationROffset=0  TranslationROffsetUnits=m  TranslationThetaOffset=0  TranslationThetaOffsetUnits=deg  TranslationZOffset=0  TranslationZOffsetUnits=m
  W2SwaRL : sm_lib/Frames and Transforms/Rigid Transform  RotationMethod=None  FollAlignAxisA=+X  BaseAlignAxisA=+Y  FollAlignAxisB=+Y  BaseAlignAxisB=+Z  RotationStandardAxis=+X  RotationAngle=-90  RotationAngleUnits=deg  RotationArbitraryAxis=[0 0 1]  RotationSequenceAxes=FollowerAxes  RotationSequence=XYX  RotationSequenceAngles=[0 0 0]  RotationSequenceAnglesUnits=deg  RotationMatrix=[1 0 0;0 1 0;0 0 1]  Quaternion=[1 0 0 0]  TranslationMethod=Cartesian  TranslationCartesianOffset=cabin.swingArmChasRL  TranslationCartesianOffsetUnits=m  TranslationStandardAxis=+Z  TranslationStandardOffset=0  TranslationStandardOffsetUnits=m  TranslationROffset=0  TranslationROffsetUnits=m  TranslationThetaOffset=0  TranslationThetaOffsetUnits=deg  TranslationZOffset=0  TranslationZOffsetUnits=m
  W2SwaRR : sm_lib/Frames and Transforms/Rigid Transform  RotationMethod=None  FollAlignAxisA=+X  BaseAlignAxisA=+Y  FollAlignAxisB=+Y  BaseAlignAxisB=+Z  RotationStandardAxis=+X  RotationAngle=-90  RotationAngleUnits=deg  RotationArbitraryAxis=[0 0 1]  RotationSequenceAxes=FollowerAxes  RotationSequence=XYX  RotationSequenceAngles=[0 0 0]  RotationSequenceAnglesUnits=deg  RotationMatrix=[1 0 0;0 1 0;0 0 1]  Quaternion=[1 0 0 0]  TranslationMethod=Cartesian  TranslationCartesianOffset=cabin.swingArmChasRR  TranslationCartesianOffsetUnits=m  TranslationStandardAxis=+Z  TranslationStandardOffset=0  TranslationStandardOffsetUnits=m  TranslationROffset=0  TranslationROffsetUnits=m  TranslationThetaOffset=0  TranslationThetaOffsetUnits=deg  TranslationZOffset=0  TranslationZOffsetUnits=m
  World : PMIOPort  Side=Left
  SwaRR : PMIOPort  Port=2  Side=Left
  SwaRL : PMIOPort  Port=3  Side=Left
  ShockRR : PMIOPort  Port=4  Side=Right
  ShockRL : PMIOPort  Port=5  Side=Right
  Cabin : PMIOPort  Port=6  Side=Right
  ShockFL : PMIOPort  Port=7  Side=Right
  ShockFR : PMIOPort  Port=8  Side=Right
  SwaFR : PMIOPort  Port=9  Side=Right
  SwaFL : PMIOPort  Port=10  Side=Right
  Bus Element Out : Outport  PortName=cabinCOG  Element=px
  BusElementOut : Outport  PortName=cabinCOG  Element=py
  BusElementOut1 : Outport  PortName=cabinCOG  Element=pz
  BusElementOut2 : Outport  PortName=cabinCOG  Element=angx
  BusElementOut3 : Outport  PortName=cabinCOG  Element=angy
  BusElementOut4 : Outport  PortName=cabinCOG  Element=angz
  wires:
  PS-Simulink Converter5/1 -> BusElementOut4/1
  PS-Simulink Converter4/1 -> BusElementOut3/1
  PS-Simulink Converter3/1 -> BusElementOut2/1
  PS-Simulink Converter2/1 -> BusElementOut1/1
  PS-Simulink Converter1/1 -> BusElementOut/1
  PS-Simulink Converter/1 -> Bus Element Out/1
  connections:
  Arrow/LConn1 -- World/RConn1 -- Initial COG/LConn1 -- "Sensor "/LConn1 -- Joint Cabin/LConn1 -- W2ShockFL/LConn1 -- W2ShockFR/LConn1 -- W2SwaFL/LConn1 -- W2SwaFR/LConn1 -- W2ShockRR/LConn1 -- W2ShockRL/LConn1 -- W2SwaRL/LConn1 -- W2SwaRR/LConn1
  W2SwaRR/RConn1 -- SwaRR/RConn1
  W2SwaRL/RConn1 -- SwaRL/RConn1
  PS-Simulink Converter5/LConn1 -- Joint Cabin/RConn4
  PS-Simulink Converter4/LConn1 -- Joint Cabin/RConn3
  PS-Simulink Converter3/LConn1 -- Joint Cabin/RConn2
  PS-Simulink Converter2/LConn1 -- "Sensor "/RConn4
  PS-Simulink Converter1/LConn1 -- "Sensor "/RConn3
  PS-Simulink Converter/LConn1 -- "Sensor "/RConn2
  Joint Cabin/RConn1 -- "Sensor "/RConn1 -- Cabin/RConn1
  W2SwaFL/RConn1 -- SwaFL/RConn1
  W2SwaFR/RConn1 -- SwaFR/RConn1
  ShockRL/RConn1 -- W2ShockRL/RConn1
  ShockRR/RConn1 -- W2ShockRR/RConn1
  ShockFL/RConn1 -- W2ShockFL/RConn1
  ShockFR/RConn1 -- W2ShockFR/RConn1

== system cabin_suspension/Shock FL ==
  Shock FL : Linkage_Shock/Shock Multibody  shock_pist_mass=cabin.shockPistonMass  shock_cyl_mass=cabin.shockCylmass  springTable=cabin.springFront  damperTable=cabin.damperFront  hp_spr_top=cabin.schockTopPosFL  hp_spr_bot=cabin.schockBotPosFL  up_lim_bumpstop=0.05  low_lim_bumpstop=-0.05  size_conn_shock=0.025  clr_shock_cyl=[0.2,0.4,0.6]  opc_shock_cyl=1  radius_shock_cyl=0.03  clr_shock_piston=[0.5,0.5,0.5]  opc_shock_piston=1  clr_shock_bumpstop=[0.93,0.93,0.56]  opc_shock_bumpstop=1  deadvol_len_shock_cyl=cabin.deadVolLength  piston_len_shock=cabin.shockPistonLength  cyl_cap_len_shock=cabin.cylCapLength  bumpstop_len_shock=cabin.bumpLength
  Cab : PMIOPort  Side=Right
  Chs : PMIOPort  Port=2  Side=Left
  tag scope: ShockFL=global
  wires:
  Shock FL/1 -> [ShockFL]  "ShockFL"
  connections:
  Chs/RConn1 -- Shock FL/LConn1
  Cab/RConn1 -- Shock FL/RConn1

== system cabin_suspension/Shock FR ==
  Shock FR : Linkage_Shock/Shock Multibody  shock_pist_mass=cabin.shockPistonMass  shock_cyl_mass=cabin.shockCylmass  springTable=cabin.springFront  damperTable=cabin.damperFront  hp_spr_top=cabin.schockTopPosFR  hp_spr_bot=cabin.schockBotPosFR  up_lim_bumpstop=0.05  low_lim_bumpstop=-0.05  size_conn_shock=0.025  clr_shock_cyl=[0.2,0.4,0.6]  opc_shock_cyl=1  radius_shock_cyl=0.03  clr_shock_piston=[0.5,0.5,0.5]  opc_shock_piston=1  clr_shock_bumpstop=[0.93,0.93,0.56]  opc_shock_bumpstop=1  deadvol_len_shock_cyl=cabin.deadVolLength  piston_len_shock=cabin.shockPistonLength  cyl_cap_len_shock=cabin.cylCapLength  bumpstop_len_shock=cabin.bumpLength
  Cab : PMIOPort  Side=Right
  Chs : PMIOPort  Port=2  Side=Left
  tag scope: ShockFR=global
  wires:
  Shock FR/1 -> [ShockFR]  "ShockFR"
  connections:
  Chs/RConn1 -- Shock FR/LConn1
  Cab/RConn1 -- Shock FR/RConn1

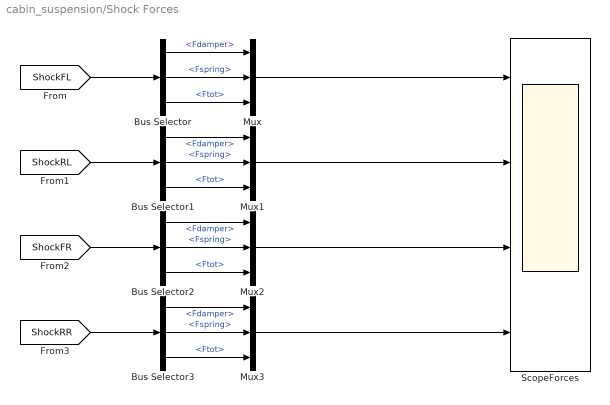
== system cabin_suspension/Shock Forces ==
  Bus Selector{,1..3} (4 alike) : BusSelector  OutputSignals=Fdamper,Fspring,Ftot
  Mux{,1..3} (4 alike) : Mux  Inputs=3
  ScopeForces : Scope  NumInputPorts=4
  wires:
  [ShockRR] -> Bus Selector3/1
  Bus Selector3/3 -> Mux3/3  "<Ftot>"
  Bus Selector3/2 -> Mux3/2  "<Fspring>"
  Mux3/1 -> ScopeForces/4
  Bus Selector3/1 -> Mux3/1  "<Fdamper>"
  [ShockFR] -> Bus Selector2/1
  Bus Selector2/3 -> Mux2/3  "<Ftot>"
  Bus Selector2/2 -> Mux2/2  "<Fspring>"
  Mux2/1 -> ScopeForces/3
  Bus Selector2/1 -> Mux2/1  "<Fdamper>"
  [ShockRL] -> Bus Selector1/1
  Bus Selector1/3 -> Mux1/3  "<Ftot>"
  Bus Selector1/2 -> Mux1/2  "<Fspring>"
  Mux1/1 -> ScopeForces/2
  Bus Selector1/1 -> Mux1/1  "<Fdamper>"
  Mux/1 -> ScopeForces/1
  Bus Selector/1 -> Mux/1  "<Fdamper>"
  Bus Selector/2 -> Mux/2  "<Fspring>"
  Bus Selector/3 -> Mux/3  "<Ftot>"
  [ShockFL] -> Bus Selector/1

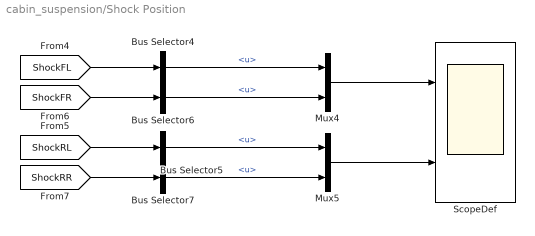
== system cabin_suspension/Shock Position ==
  Bus Selector{4..7} (4 alike) : BusSelector  OutputSignals=u
  Mux4 : Mux  Inputs=2
  Mux5 : Mux  Inputs=2
  ScopeDef : Scope  NumInputPorts=2
  wires:
  Bus Selector5/1 -> Mux5/1  "<u>"
  Bus Selector7/1 -> Mux5/2  "<u>"
  Mux5/1 -> ScopeDef/2
  [ShockRR] -> Bus Selector7/1
  [ShockRL] -> Bus Selector5/1
  [ShockFR] -> Bus Selector6/1
  Bus Selector6/1 -> Mux4/2  "<u>"
  Mux4/1 -> ScopeDef/1
  Bus Selector4/1 -> Mux4/1  "<u>"
  [ShockFL] -> Bus Selector4/1

== system cabin_suspension/Shock RL ==
  Shock RL : Linkage_Shock/Shock Multibody  shock_pist_mass=cabin.shockPistonMass  shock_cyl_mass=cabin.shockCylmass  springTable=cabin.springRear  damperTable=cabin.damperRear  hp_spr_top=cabin.schockTopPosRL  hp_spr_bot=cabin.schockBotPosRL  up_lim_bumpstop=0.05  low_lim_bumpstop=-0.05  size_conn_shock=0.025  clr_shock_cyl=[0.2,0.4,0.6]  opc_shock_cyl=1  radius_shock_cyl=0.03  clr_shock_piston=[0.5,0.5,0.5]  opc_shock_piston=1  clr_shock_bumpstop=[0.93,0.93,0.56]  opc_shock_bumpstop=1  deadvol_len_shock_cyl=cabin.deadVolLength  piston_len_shock=cabin.shockPistonLength  cyl_cap_len_shock=cabin.cylCapLength  bumpstop_len_shock=cabin.bumpLength
  Cab : PMIOPort  Side=Right
  Chs : PMIOPort  Port=2  Side=Left
  tag scope: ShockRL=global
  wires:
  Shock RL/1 -> [ShockRL]  "ShockRL"
  connections:
  Chs/RConn1 -- Shock RL/LConn1
  Cab/RConn1 -- Shock RL/RConn1

== system cabin_suspension/Shock RR ==
  Shock RR : Linkage_Shock/Shock Multibody  shock_pist_mass=cabin.shockPistonMass  shock_cyl_mass=cabin.shockCylmass  springTable=cabin.springRear  damperTable=cabin.damperRear  hp_spr_top=cabin.schockTopPosRR  hp_spr_bot=cabin.schockBotPosRR  up_lim_bumpstop=0.05  low_lim_bumpstop=-0.05  size_conn_shock=0.025  clr_shock_cyl=[0.2,0.4,0.6]  opc_shock_cyl=1  radius_shock_cyl=0.03  clr_shock_piston=[0.5,0.5,0.5]  opc_shock_piston=1  clr_shock_bumpstop=[0.93,0.93,0.56]  opc_shock_bumpstop=1  deadvol_len_shock_cyl=cabin.deadVolLength  piston_len_shock=cabin.shockPistonLength  cyl_cap_len_shock=cabin.cylCapLength  bumpstop_len_shock=cabin.bumpLength
  Cab : PMIOPort  Side=Right
  Chs : PMIOPort  Port=2  Side=Left
  tag scope: ShockRR=global
  wires:
  Shock RR/1 -> [ShockRR]  "ShockRR"
  connections:
  Cab/RConn1 -- Shock RR/RConn1
  Chs/RConn1 -- Shock RR/LConn1

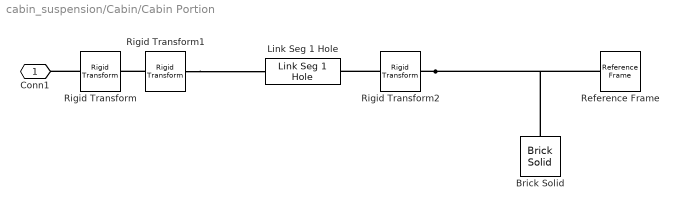
== system cabin_suspension/Cabin/Cabin Portion ==
  Brick Solid : sm_lib/Body Elements/Brick Solid  BrickDimensions=[0.01 cabin.schockTopPosFL(1) cabin.schockTopPosFL(2)+0.005]  BrickDimensionsUnits=m  ExportEntireGeometry=off  InertiaType=PointMass  BasedOnType=Density  Density=1000  DensityUnits=kg/m^3  Mass=0  MassUnits=kg  CenterOfMass=[0 0 0]  CenterOfMassUnits=m  MomentsOfInertia=[1 1 1]  MomentsOfInertiaUnits=kg*m^2  ProductsOfInertia=[0 0 0]  ProductsOfInertiaUnits=kg*m^2  GraphicType=FromGeometry  MarkerShape=Sphere  MarkerSize=10  GraphicVisPropType=SimpleVisualProperties  GraphicDiffuseColor=cabin.cabinColor  GraphicOpacity=cabin.cabinOpacity  GraphicSpecularColor=[0.5 0.5 0.5 1.0]  GraphicAmbientColor=[0.15 0.15 0.15 1.0]  GraphicEmissiveColor=[0.0 0.0 0.0 1.0]  GraphicShininess=75  DoExposeReferenceFrame=off  SerializedFrames=<Frames><Frame><Id>Frame1</Id><Value><Name>F1</Name><Origin><Source>GeometricFeature</Source><FeatureName>-x -y -z point</FeatureName></Origin><PrimaryAxis><DefinedDirection>+Z</DefinedDirection><Source>ReferenceFrame</Source><SourceDirection>+Z</SourceDirection><FeatureName></FeatureName></PrimaryAxis><SecondaryAxis><DefinedDirection>-Y</DefinedDirection><Source>ReferenceFrame</Source><SourceDirection>+Y</SourceDirection><FeatureName></FeatureName></SecondaryAxis></Value></Frame></Frames>
  Link Seg 1 Hole : Linkage_Shock/Link Seg 1 Hole  link_len=0.65-cabin.schockTopPosFL(3)  link_width=0.05  link_radh=0.005  link_holelr=+X  link_thickness=0.01  link_rho=0  link_color=cabin.cabinColor  link_opc=cabin.cabinOpacity
  Reference Frame : sm_lib/Frames and Transforms/Reference Frame
  Rigid Transform : sm_lib/Frames and Transforms/Rigid Transform  RotationMethod=StandardAxis  FollAlignAxisA=+X  BaseAlignAxisA=+Y  FollAlignAxisB=+Y  BaseAlignAxisB=+Z  RotationStandardAxis=+Y  RotationAngle=90  RotationAngleUnits=deg  RotationArbitraryAxis=[0 0 1]  RotationSequenceAxes=FollowerAxes  RotationSequence=XYX  RotationSequenceAngles=[0 0 0]  RotationSequenceAnglesUnits=deg  RotationMatrix=[1 0 0;0 1 0;0 0 1]  Quaternion=[1 0 0 0]  TranslationMethod=None  TranslationCartesianOffset=[0 0 0]  TranslationCartesianOffsetUnits=m  TranslationStandardAxis=+Z  TranslationStandardOffset=0  TranslationStandardOffsetUnits=m  TranslationROffset=0  TranslationROffsetUnits=m  TranslationThetaOffset=0  TranslationThetaOffsetUnits=deg  TranslationZOffset=0  TranslationZOffsetUnits=m
  Rigid Transform1 : sm_lib/Frames and Transforms/Rigid Transform  RotationMethod=StandardAxis  FollAlignAxisA=+X  BaseAlignAxisA=+Y  FollAlignAxisB=+Y  BaseAlignAxisB=+Z  RotationStandardAxis=+X  RotationAngle=90  RotationAngleUnits=deg  RotationArbitraryAxis=[0 0 1]  RotationSequenceAxes=FollowerAxes  RotationSequence=XYX  RotationSequenceAngles=[0 0 0]  RotationSequenceAnglesUnits=deg  RotationMatrix=[1 0 0;0 1 0;0 0 1]  Quaternion=[1 0 0 0]  TranslationMethod=None  TranslationCartesianOffset=[0 0 0]  TranslationCartesianOffsetUnits=m  TranslationStandardAxis=+Z  TranslationStandardOffset=0  TranslationStandardOffsetUnits=m  TranslationROffset=0  TranslationROffsetUnits=m  TranslationThetaOffset=0  TranslationThetaOffsetUnits=deg  TranslationZOffset=0  TranslationZOffsetUnits=m
  Rigid Transform2 : sm_lib/Frames and Transforms/Rigid Transform  RotationMethod=None  FollAlignAxisA=+X  BaseAlignAxisA=+Y  FollAlignAxisB=+Y  BaseAlignAxisB=+Z  RotationStandardAxis=+Z  RotationAngle=0  RotationAngleUnits=deg  RotationArbitraryAxis=[0 0 1]  RotationSequenceAxes=FollowerAxes  RotationSequence=XYX  RotationSequenceAngles=[0 0 0]  RotationSequenceAnglesUnits=deg  RotationMatrix=[1 0 0;0 1 0;0 0 1]  Quaternion=[1 0 0 0]  TranslationMethod=Cartesian  TranslationCartesianOffset=[0, abs(cabin.schockBotPosFL(1)-cabin.swingArmCabFL(1))+0.025, -0.005]  TranslationCartesianOffsetUnits=m  TranslationStandardAxis=+Z  TranslationStandardOffset=0  TranslationStandardOffsetUnits=m  TranslationROffset=0  TranslationROffsetUnits=m  TranslationThetaOffset=0  TranslationThetaOffsetUnits=deg  TranslationZOffset=0  TranslationZOffsetUnits=m
  Conn1 : PMIOPort  Side=Left
  connections:
  Rigid Transform2/LConn1 -- Link Seg 1 Hole/LConn1
  Rigid Transform2/RConn1 -- Brick Solid/LConn1 -- Reference Frame/RConn1
  Rigid Transform/LConn1 -- Conn1/RConn1
  Rigid Transform1/RConn1 -- Link Seg 1 Hole/RConn1
  Rigid Transform1/LConn1 -- Rigid Transform/RConn1

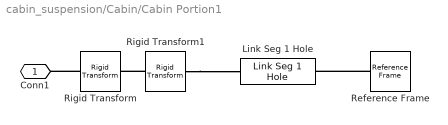
== system cabin_suspension/Cabin/Cabin Portion1 ==
  Link Seg 1 Hole : Linkage_Shock/Link Seg 1 Hole  link_len=0.65-cabin.swingArmCabFL(3)  link_width=0.05  link_radh=0.005  link_holelr=+X  link_thickness=0.01  link_rho=0  link_color=cabin.cabinColor  link_opc=cabin.cabinOpacity
  Reference Frame : sm_lib/Frames and Transforms/Reference Frame
  Rigid Transform : sm_lib/Frames and Transforms/Rigid Transform  RotationMethod=StandardAxis  FollAlignAxisA=+X  BaseAlignAxisA=+Y  FollAlignAxisB=+Y  BaseAlignAxisB=+Z  RotationStandardAxis=+Y  RotationAngle=90  RotationAngleUnits=deg  RotationArbitraryAxis=[0 0 1]  RotationSequenceAxes=FollowerAxes  RotationSequence=XYX  RotationSequenceAngles=[0 0 0]  RotationSequenceAnglesUnits=deg  RotationMatrix=[1 0 0;0 1 0;0 0 1]  Quaternion=[1 0 0 0]  TranslationMethod=None  TranslationCartesianOffset=[0 0 0]  TranslationCartesianOffsetUnits=m  TranslationStandardAxis=+Z  TranslationStandardOffset=0  TranslationStandardOffsetUnits=m  TranslationROffset=0  TranslationROffsetUnits=m  TranslationThetaOffset=0  TranslationThetaOffsetUnits=deg  TranslationZOffset=0  TranslationZOffsetUnits=m
  Rigid Transform1 : sm_lib/Frames and Transforms/Rigid Transform  RotationMethod=StandardAxis  FollAlignAxisA=+X  BaseAlignAxisA=+Y  FollAlignAxisB=+Y  BaseAlignAxisB=+Z  RotationStandardAxis=+X  RotationAngle=90  RotationAngleUnits=deg  RotationArbitraryAxis=[0 0 1]  RotationSequenceAxes=FollowerAxes  RotationSequence=XYX  RotationSequenceAngles=[0 0 0]  RotationSequenceAnglesUnits=deg  RotationMatrix=[1 0 0;0 1 0;0 0 1]  Quaternion=[1 0 0 0]  TranslationMethod=None  TranslationCartesianOffset=[0 0 0]  TranslationCartesianOffsetUnits=m  TranslationStandardAxis=+Z  TranslationStandardOffset=0  TranslationStandardOffsetUnits=m  TranslationROffset=0  TranslationROffsetUnits=m  TranslationThetaOffset=0  TranslationThetaOffsetUnits=deg  TranslationZOffset=0  TranslationZOffsetUnits=m
  Conn1 : PMIOPort  Side=Left
  connections:
  Reference Frame/RConn1 -- Link Seg 1 Hole/LConn1
  Rigid Transform/LConn1 -- Conn1/RConn1
  Rigid Transform1/RConn1 -- Link Seg 1 Hole/RConn1
  Rigid Transform1/LConn1 -- Rigid Transform/RConn1
